simulink library "MidSideLibrary_Solution"  (R2024b)
settings: Solver=VariableStepAuto  StartTime=0.0  StopTime=10.0  RelTol=1e-3
settings Model: Creator=skerber  LastModifiedBy=skerber

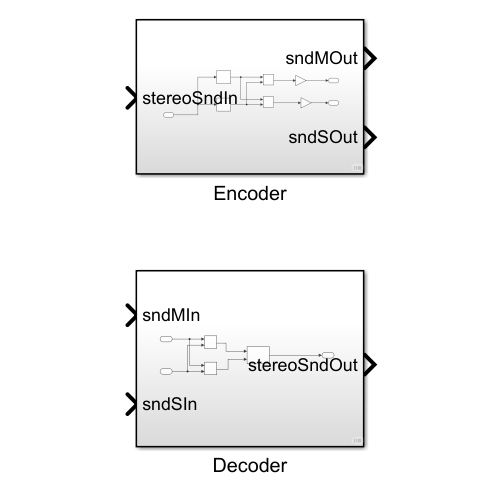
[thumbnail: Simulink's stored preview of the top-level diagram]
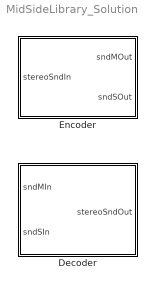
== system MidSideLibrary_Solution ==
  Decoder : Subsystem
  Encoder : Subsystem

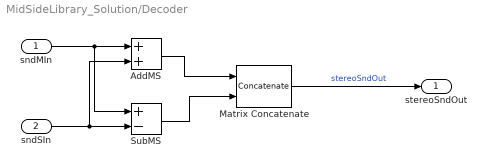
== system MidSideLibrary_Solution/Decoder ==
  sndMIn : Inport
  sndSIn : Inport  Port=2
  AddMS : Sum
  Matrix Concatenate : Concatenate  Mode=Multidimensional array  ConcatenateDimension=2
  SubMS : Sum  Inputs=+-
  stereoSndOut : Outport
  wires:
  SubMS/1 -> Matrix Concatenate/2
  sndSIn/1 -> SubMS/2, AddMS/2
  Matrix Concatenate/1 -> stereoSndOut/1  "stereoSndOut"
  AddMS/1 -> Matrix Concatenate/1
  sndMIn/1 -> AddMS/1, SubMS/1

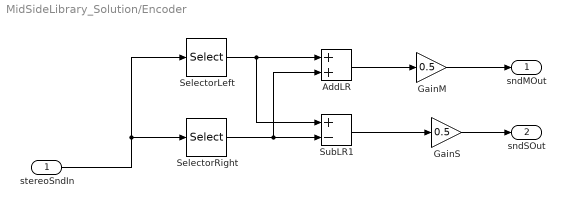
== system MidSideLibrary_Solution/Encoder ==
  stereoSndIn : Inport
  AddLR : Sum
  GainM : Gain  Gain=0.5
  GainS : Gain  Gain=0.5
  SelectorLeft : Selector  NumberOfDimensions=2  InputPortWidth=3  IndexOptions=Select all,Index vector (dialog)  Indices=[1 3],1  OutputSizes=1,1
  SelectorRight : Selector  NumberOfDimensions=2  InputPortWidth=3  IndexOptions=Select all,Index vector (dialog)  Indices=[1 3],2  OutputSizes=1,1
  SubLR1 : Sum  Inputs=+-
  sndMOut : Outport
  sndSOut : Outport  Port=2
  wires:
  SelectorRight/1 -> AddLR/2, SubLR1/2
  SubLR1/1 -> GainS/1
  GainM/1 -> sndMOut/1
  AddLR/1 -> GainM/1
  stereoSndIn/1 -> SelectorRight/1, SelectorLeft/1
  GainS/1 -> sndSOut/1
  SelectorLeft/1 -> AddLR/1, SubLR1/1
